simulink library "tp333079"  (Simulink 5.0)
values from neighbouring files (symbols this model uses):
  b = 1    [main_flock3.m]    (also in main_flock4.m; params_flocking_ros.m)
undefined symbols (not defined in the file or in its folder): AC, AlphaBnd, BetaBnd, CDda, CDde, CDdf, CDdr, CDM, CDmin, CGempty, CGgross, CL0, CLa, CLalphadot, Clbeta, Clda, CLde, CLdf, Cldr, CLM, CLmind, Clp, CLq, Clr, Cm0, Cma, Cmalphadot, Cmde, Cmdf, CmM, Cmq, Cnbeta, Cnda, Cndr, Cnp, Cnr, CP, CT, CYbeta, CYda, CYdr, CYp, CYr, Displacement, dmy, Engine, EulerIni, FuelFlow, FuelIni, J, Jempty, Jeng, Jgross, Jprop, MAC, MAP, MAPLim, MassIni, MaxPower, mempty ... (+26)
libraries: aerosimlib x325, simulink3 x42
(part 1 of 11)
Description:
  | AeroSim Aircraft Simulation Library
settings Model: Creator=Marius Niculescu  LastModifiedBy=mariusn

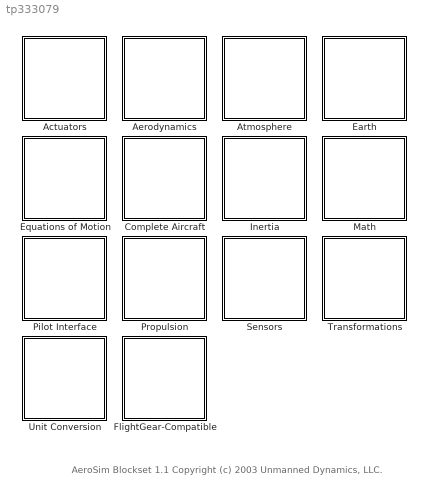
== system tp333079 ==
  note: AeroSim Blockset 1.1
      | Copyright (c) 2003 Unmanned Dynamics, LLC.
  Actuators : Subsystem  SimViewingDevice=off
      settings: Permissions=ReadWrite  RTWFcnNameOpts=Auto  RTWFileNameOpts=Auto
      mask Display: image(imread('act.bmp','bmp'))
  Aerodynamics : Subsystem  SimViewingDevice=off
      settings: Permissions=ReadWrite  RTWFcnNameOpts=Auto  RTWFileNameOpts=Auto
      mask Display: image(imread('aero.bmp','bmp'))
  Atmosphere : Subsystem  SimViewingDevice=off
      settings: Permissions=ReadWrite  RTWFcnNameOpts=Auto  RTWFileNameOpts=Auto
      mask Display: image(imread('atmo.bmp','bmp'))
  Complete Aircraft : Subsystem  SimViewingDevice=off
      settings: Permissions=ReadWrite  RTWFcnNameOpts=Auto  RTWFileNameOpts=Auto
      mask Display: image(imread('sample.bmp','bmp'))
  Earth : Subsystem  SimViewingDevice=off
      settings: Permissions=ReadWrite  RTWFcnNameOpts=Auto  RTWFileNameOpts=Auto
      mask Display: image(imread('earth.bmp','bmp'))
  Equations of Motion : Subsystem  SimViewingDevice=off
      settings: Permissions=ReadWrite  RTWFcnNameOpts=Auto  RTWFileNameOpts=Auto
      mask Display: image(imread('eom.bmp','bmp'))
  FlightGear-Compatible : Subsystem  SimViewingDevice=off
      settings: Permissions=ReadWrite  RTWFcnNameOpts=Auto  RTWFileNameOpts=Auto
      mask Display: image(imread('fg.bmp','bmp'))
  Inertia : Subsystem  SimViewingDevice=off
      settings: Permissions=ReadWrite  RTWFcnNameOpts=Auto  RTWFileNameOpts=Auto
      mask Display: image(imread('inertia.bmp','bmp'))
  Math : Subsystem  SimViewingDevice=off
      settings: Permissions=ReadWrite  RTWFcnNameOpts=Auto  RTWFileNameOpts=Auto
      mask Display: image(imread('linalg.bmp','bmp'))
  Pilot Interface : Subsystem  SimViewingDevice=off
      settings: Permissions=ReadWrite  RTWFcnNameOpts=Auto  RTWFileNameOpts=Auto
      mask Display: image(imread('pilot.bmp','bmp'))
  Propulsion : Subsystem  SimViewingDevice=off
      settings: Permissions=ReadWrite  RTWFcnNameOpts=Auto  RTWFileNameOpts=Auto
      mask Display: image(imread('prop.bmp','bmp'))
  Sensors : Subsystem  SimViewingDevice=off
      settings: Permissions=ReadWrite  RTWFcnNameOpts=Auto  RTWFileNameOpts=Auto
      mask Display: image(imread('sensor.bmp','bmp'))
  Transformations : Subsystem  SimViewingDevice=off
      settings: Permissions=ReadWrite  RTWFcnNameOpts=Auto  RTWFileNameOpts=Auto
      mask Display: image(imread('transf.bmp','bmp'))
  Unit Conversion : Subsystem  SimViewingDevice=off
      settings: Permissions=ReadWrite  RTWFcnNameOpts=Auto  RTWFileNameOpts=Auto
      mask Display: image(imread('units.bmp','bmp'))

== system tp333079/Actuators ==
  D/A Converter : Subsystem  SimViewingDevice=off  mask(D/A Converter){Vrange=[0 5], Bits=10, tsamp=0.02}
      mask prompts: Vrange "Voltage range [min max]:"; Bits "Resolution [bits]:"; tsamp "Sample time [s]:"
      mask help: Convert the digital signal with the specified resolution to analog voltage within a specified voltage range.
      mask init:
      | MinVolts = Vrange(1);
      | MaxVolts = Vrange(2);
      settings: Permissions=ReadWrite  RTWFcnNameOpts=Auto  RTWFileNameOpts=Auto
      mask Help:
      | <P>The D/A converter accepts a discrete signal as an integer number (counts) for input and provides an analog voltage. The parameters that have to be set are the following:</P>
      | <LI>Voltage range = a 1x2 vector with the minimum and maximum values of the output voltage;</LI>
      | <LI>Resolution = the maximum number of counts for input, i.e. a 10-bit converter can output maximum 2^10 = 1024 counts;</LI>
      | <LI>Sample time = input count update rate.</LI>
  Simple Actuator (1st-order dynamics) : Subsystem  SimViewingDevice=off  mask(Simple actuator){MaxRate=0.1, CountRange=[0 1024], ActRange=[-1 1], Lag=0.01}
      mask prompts: MaxRate "Max actuation rate:"; CountRange "Input signal range [min max]:"; ActRange "Actuator range [min max]:"; Lag "Actuator lag:"
      mask help: Simple actuator featuring 1st order dynamics, saturation and rate limits.
      mask init:
      | MinAct = ActRange(1); MaxAct = ActRange(2);
      | MinCounts = CountRange(1); MaxCounts = CountRange(2);
      settings: Permissions=ReadWrite  RTWFcnNameOpts=Auto  RTWFileNameOpts=Auto
      mask Help:
      | The block provides a simple actuator model which includes scaling, linear dynamics, saturation, and rate limits.
      | <P><B>Parameters:</B>
      | <LI>Maximum actuation rate = the max actuator travel speed, (travel per second)</LI>
      | <LI>Input signal range = the 1x2 vector which includes the min and max values of the input signal (for example, for a 10-bit analog output signal, the range would be [0 1023]).</LI>
      | <LI>Actuator range = the actuator travel range.</LI>
      | <LI>Actuator lag = the time lag of the actuator output.</LI>
      | </P>
  Simple Actuator (2nd-order dynamics) : Subsystem  SimViewingDevice=off  mask(Simple actuator){MaxRate=0.1, CountRange=[0 1024], ActRange=[-1 1], Bandwidth=100}
      mask prompts: MaxRate "Max actuation rate:"; CountRange "Input signal range [min max]:"; ActRange "Actuator range [min max]:"; Bandwidth "Bandwidth at -3dB [Hz]:"
      mask help: Simple actuator featuring 2nd order dynamics, saturation and rate limits.
      mask init:
      | MinAct = ActRange(1); MaxAct = ActRange(2);
      | MinCounts = CountRange(1); MaxCounts = CountRange(2);
      | wn = 2*pi*Bandwidth;
      | zeta = 0.5*10^(3/20);
      settings: Permissions=ReadWrite  RTWFcnNameOpts=Auto  RTWFileNameOpts=Auto
      mask Help:
      | The block provides a simple actuator model which includes scaling, linear dynamics, saturation, and rate limits.
      | <P><B>Parameters:</B>
      | <LI>Maximum actuation rate = the max actuator travel speed, (travel per second)</LI>
      | <LI>Input signal range = the 1x2 vector which includes the min and max values of the input signal (for example, for a 10-bit analog output signal, the range would be [0 1023]).</LI>
      | <LI>Actuator range = the actuator travel range.</LI>
      | <LI>Bandwidth at -3dB = the actuator bandwidth at -90 deg phase and -3dB gain.</LI>
      | </P>
  wires:
  Simple Actuator (2nd-order dynamics)/1(Output) -> ?

== system tp333079/Aerodynamics ==
  Aerodynamic Force : Subsystem  SimViewingDevice=off  mask(Aerodynamic force){S=S}
      mask prompts: S "Wing reference area:"
      mask help: Computes aerodynamic force in body axes.
      settings: Permissions=ReadWrite  RTWFcnNameOpts=Auto  RTWFileNameOpts=Auto
      mask Help:
      | The block computes the aerodynamic force in body axes.
      | <P><B>Inputs:</B>
      | <LI>CD = the coefficient of drag</LI>
      | <LI>CY = the coefficient of side force</LI>
      | <LI>CL = the coefficient of lift</LI>
      | <LI>pdyn = the dynamic pressure</LI>
      | <LI>WindAxesVel = the 3x1 vector of wind axes velocity components [Va beta alpha]'</LI>
      | </P>
      | <P><B>Output:</B> the 3x1 vector of aerodynamic forces in body axes</P>
      | <P><B>Parameters:</B>
      | <LI>S = the wing reference area</LI>
      | </P>
  Aerodynamic Moment : Subsystem  SimViewingDevice=off  mask(Aerodynamic moment){c=MAC, b=b, S=S}
      mask prompts: c "Mean aerodynamic chord:"; b "Wing span:"; S "Wing reference area:"
      mask help: Computes aerodynamic moment with respect to the aerodynamic center.
      settings: Permissions=ReadWrite  RTWFcnNameOpts=Auto  RTWFileNameOpts=Auto
      mask Help:
      | The block computes the aerodynamic moment with respect to the aerodynamic center.
      | <P><B>Inputs:</B>
      | <LI>Cl = the roll moment coefficient</LI>
      | <LI>Cm = the pitch moment coefficient</LI>
      | <LI>Cn = the yaw moment coefficient</LI>
      | </P>
      | <P><B>Output:</B> the 3x1 vector of aerodynamic moments about the aerodynamic center</P>
      | <P><B>Parameters:</B>
      | <LI>c = the mean aerodynamic chord</LI>
      | <LI>b = the reference wing span</LI>
      | <LI>S = the reference wing area</LI>
      | </P>
  Drag Coefficient : Subsystem  SimViewingDevice=off  mask(Drag coefficient){CL0=CLmind, CD0=CDmin, CDdf=CDdf, CDde=CDde, CDda=CDda, CDdr=CDdr, CDM=CDM, e=osw, b=b, S=S}
      mask prompts: CL0 "Lift at minimum drag (CL0):"; CD0 "Minimum drag (CD0):"; CDdf "Lift control derivative (CDdf):"; CDde "Pitch control derivative (CDde):"; CDda "Roll control derivative (CDda):"; CDdr "Yaw control derivative (CDdr):"; CDM "Mach number derivative (CDM):"; e "Oswald's coefficient (e):"; b "Wing span (b):"; S "Wing reference area (S):"
      mask help: Computes the drag coefficient by linear component build-up.
      mask init:
      | AR = b^2/S;
      | k = 1/(pi*AR*e);
      settings: Permissions=ReadWrite  RTWFcnNameOpts=Auto  RTWFileNameOpts=Auto
      mask Help:
      | The block computes the airplane drag coefficient using linear component build-up method.
      | <P><B>Inputs:</B>
      | <LI>WindAxesVel = the 3x1 vector of wind axes velocity components [Va beta alpha]'</LI>
      | <LI>Control = the 4x1 vector of aerodynamic controls [Flap Elevator Aileron Rudder]'</LI>
      | <LI>CL = the current coefficient of lift</LI>
      | <LI>Mach = the Mach number.</LI>
      | </P>
      | <P><B>Output:</B> the coefficient of drag CD.</P>
      | <P><B>Parameters:</B>
      | <LI>CL0 = CL at minimum drag</LI>
      | <LI>CD0 = minimum drag</LI>
      | <LI>CDdf = CD sensitivity to flap deflection</LI>
      | <LI>CDde = CD sensitivity to elevator deflection</LI>
      | <LI>CDda = CD sensitivity to aileron deflection</LI>
      | <LI>CDdr = CD sensitivity to rudder deflection</LI>
      | <LI>CDM = CD sensitivity to Mach number</LI>
      | <LI>e = the Oswald coefficient, for induced drag</LI>
      | <LI>b = the reference span</LI>
      | <LI>S = the reference area</LI>
      | </P>
  Dynamic Pressure : Subsystem  SimViewingDevice=off
      settings: Permissions=ReadWrite  RTWFcnNameOpts=Auto  RTWFileNameOpts=Auto
      mask Type: Dynamic pressure
      mask Description: Computes dynamic pressure based on current airspeed and air density.
      mask Help:
      | The block computes the dynamic pressure.
      | <P><B>Inputs:</B>
      | <LI>WindAxesVel = the 3x1 vector of wind axes velocity components [Va beta alpha]'</LI>
      | <LI>rho = the air density at current altitude</LI>
      | </P>
      | <P><B>Output:</B> Dynamic pressure.</P>
  Lift Coefficient : Subsystem  SimViewingDevice=off  mask(Lift coefficient){CL0=CL0, CLalpha=CLa, CLdf=CLdf, CLde=CLde, CLalphadot=CLalphadot, CLq=CLq, CLM=CLM, c=MAC}
      mask prompts: CL0 "Zero-alpha lift (CL0):"; CLalpha "alpha derivative (CLa):"; CLdf "Lift control derivative (CLdf):"; CLde "Pitch control derivative (CLde):"; CLalphadot "alpha_dot derivative (CLalphadot):"; CLq "Pitch rate derivative (CLq):"; CLM "Mach number derivative (CLM):"; c "Mean aerodynamic chord (c):"
      mask help: Computes lift coefficient using linear component build-up.
      settings: Permissions=ReadWrite  RTWFcnNameOpts=Auto  RTWFileNameOpts=Auto
      mask Help:
      | The block computes the airplane lift coefficient using linear component build-up method.
      | <P><B>Inputs:</B>
      | <LI>WindAxesVel = the 3x1 vector of wind axes velocity components [Va beta alpha]'</LI>
      | <LI>Control = the 4x1 vector of aerodynamic controls [Flap Elevator Aileron Rudder]'</LI>
      | <LI>AlphaBetaDot = the 2x1 vector of aerodynamic angle derivatives [dalpha/dt dbeta/dt]'</LI>
      | <LI>AngularRates = the 3x1 vector of body angular rates [p q r]'</LI>
      | <LI>Mach = the Mach number.</LI>
      | </P>
      | <P><B>Output:</B> the coefficient of lift CL.</P>
      | <P><B>Parameters:</B>
      | <LI>CL0 = CL at zero angle-of-attack</LI>
      | <LI>CLa = CL sensitivity to angle of attack</LI>
      | <LI>CLdf = CL sensitivity to flap deflection</LI>
      | <LI>CLde = CL sensitivity to elevator deflection</LI>
      | <LI>CLalphadot = CL sensitivity to time variations in angle of attack</LI>
      | <LI>CLq = CL sensitivity to pitch rate</LI>
      | <LI>CLM = CL sensitivity to Mach number</LI>
      | <LI>c = the reference chord (typically the mean aerodynamic chord of the wing)</LI>
      | </P>
  Pitch Moment Coefficient : Subsystem  SimViewingDevice=off  mask(Pitch moment coefficient){Cm0=Cm0, Cma=Cma, Cmdf=Cmdf, Cmde=Cmde, Cmalphadot=Cmalphadot, Cmq=Cmq, CmM=CmM, c=MAC}
      mask prompts: Cm0 "Zero-alpha pitch (Cm0):"; Cma "alpha derivative (Cma):"; Cmdf "Lift control derivative (Cmdf):"; Cmde "Pitch control derivative (Cmde):"; Cmalphadot "alpha_dot derivative (Cmalphadot):"; Cmq "Pitch rate derivative (Cmq):"; CmM "Mach number derivative (CmM):"; c "Mean aerodynamic chord (c):"
      mask help: Computes pitch moment coefficient using linear component build-up.
      settings: Permissions=ReadWrite  RTWFcnNameOpts=Auto  RTWFileNameOpts=Auto
      mask Help:
      | The block computes the airplane pitch moment coefficient using linear component build-up method.
      | <P><B>Inputs:</B>
      | <LI>WindAxesVel = the 3x1 vector of wind axes velocity components [Va beta alpha]'</LI>
      | <LI>Control = the 4x1 vector of aerodynamic controls [Flap Elevator Aileron Rudder]'</LI>
      | <LI>AlphaBetaDot = the 2x1 vector of aerodynamic angle derivatives [dalpha/dt dbeta/dt]'</LI>
      | <LI>AngularRates = the 3x1 vector of body angular rates [p q r]'</LI>
      | <LI>Mach = the Mach number.</LI>
      | </P>
      | <P><B>Output:</B> the pitch moment coefficient Cm.</P>
      | <P><B>Parameters:</B>
      | <LI>Cm0 = Cm at zero angle-of-attack</LI>
      | <LI>Cma = Cm sensitivity to angle of attack</LI>
      | <LI>Cmdf = Cm sensitivity to flap deflection</LI>
      | <LI>Cmde = Cm sensitivity to elevator deflection</LI>
      | <LI>Cmalphadot = Cm sensitivity to time variations in angle of attack</LI>
      | <LI>Cmq = Cm sensitivity to pitch rate</LI>
      | <LI>CmM = Cm sensitivity to Mach number</LI>
      | <LI>c = the reference chord (typically the mean aerodynamic chord of the wing)</LI>
      | </P>
  Roll Moment Coefficient : Subsystem  SimViewingDevice=off  mask(Roll moment coefficient){Clbeta=Clbeta, Clda=Clda, Cldr=Cldr, Clp=Clp, Clr=Clr, b=b}
      mask prompts: Clbeta "Sideslip derivative (Clbeta):"; Clda "Roll control derivative (Clda):"; Cldr "Yaw control derivative (Cldr):"; Clp "Roll rate derivative (Clp):"; Clr "Yaw rate derivative (Clr):"; b "Wing span (b):"
      mask help: Computes the roll moment coefficient using linear aerodynamic component build-up.
      settings: Permissions=ReadWrite  RTWFcnNameOpts=Auto  RTWFileNameOpts=Auto
      mask Help:
      | The block computes the airplane roll coefficient using linear component build-up method.
      | <P><B>Inputs:</B>
      | <LI>WindAxesVel = the 3x1 vector of wind axes velocity components [Va beta alpha]'</LI>
      | <LI>Control = the 4x1 vector of aerodynamic controls [Flap Elevator Aileron Rudder]'</LI>
      | <LI>AngularRates = the 3x1 vector of body angular rates [p q r]'</LI>
      | </P>
      | <P><B>Output:</B> the roll moment coefficient Cl.</P>
      | <P><B>Parameters:</B>
      | <LI>Clbeta = Cl sensitivity to sideslip</LI>
      | <LI>Clda = Cl sensitivity to aileron deflection</LI>
      | <LI>Cldr = Cl sensitivity to rudder deflection</LI>
      | <LI>Clp = Cl sensitivity to roll rate</LI>
      | <LI>Clr = Cl sensitivity to yaw rate</LI>
      | <LI>b = the reference wing span</LI>
      | </P>
  Side Force Coefficient : Subsystem  SimViewingDevice=off  mask(Side force coefficient){CYbeta=CYbeta, CYda=CYda, CYdr=CYdr, CYp=CYp, CYr=CYr, b=b}
      mask prompts: CYbeta "Sideslip derivative (CYbeta):"; CYda "Roll control derivative (CYda):"; CYdr "Yaw control derivative (CYdr):"; CYp "Roll rate derivative (CYp):"; CYr "Yaw rate derivative (CYr):"; b "Wing span (b):"
      mask help: Computes the side force coefficient using linear aerodynamic component build-up.
      settings: Permissions=ReadWrite  RTWFcnNameOpts=Auto  RTWFileNameOpts=Auto
      mask Help:
      | The block computes the airplane side force coefficient using linear component build-up method.
      | <P><B>Inputs:</B>
      | <LI>WindAxesVel = the 3x1 vector of wind axes velocity components [Va beta alpha]'</LI>
      | <LI>Control = the 4x1 vector of aerodynamic controls [Flap Elevator Aileron Rudder]'</LI>
      | <LI>AngularRates = the 3x1 vector of body angular rates [p q r]'</LI>
      | </P>
      | <P><B>Output:</B> the coefficient of side force CY.</P>
      | <P><B>Parameters:</B>
      | <LI>CYbeta = CY sensitivity to sideslip</LI>
      | <LI>CYda = CY sensitivity to aileron deflection</LI>
      | <LI>CYdr = CY sensitivity to rudder deflection</LI>
      | <LI>CYp = CY sensitivity to roll rate</LI>
      | <LI>CYr = CY sensitivity to yaw rate</LI>
      | <LI>b = the reference wing span</LI>
      | </P>
  Wind-axes Velocities : Subsystem  SimViewingDevice=off  mask(Wind-axes velocities){Vabnd=VaBnd, betabnd=BetaBnd, alphabnd=AlphaBnd}
      mask prompts: Vabnd "Airspeed bounds [min max]:"; betabnd "Sideslip angle bounds [min max]:"; alphabnd "Angle-of-attack bounds [min max]:"
      mask help: Returns the airspeed, sideslip angle, angle-of-attack and Mach number as functions of groundspeed, winds and local speed of sound. It also computes the time derivatives of the aerodynamic angles.
      settings: Permissions=ReadWrite  RTWFcnNameOpts=Auto  RTWFileNameOpts=Auto
      mask Help:
      | The block computes the wind-axes parameters including airspeed, angle-of-attack, and sideslip, as well as the wind angles time derivatives. In addition to that, the Mach number is computed.
      | <P><B>Inputs:</B>
      | <LI>Vbody = the 3x1 vector of body velocities (these are ground speed components in body axes)</LI>
      | <LI>Wbody = the 3x1 vector of wind velocities in body axes</LI>
      | <LI>SoundSpd = the speed of sound at current altitude</LI>
      | </P>
      | <P><B>Outputs:</B>
      | <LI>WindAxesVel = the 3x1 vector of wind-axes velocities [Va beta alpha]'</LI>
      | <LI>AlphaBetaDot = the 2x1 vector of angle derivatives [dalpha/dt dbeta/dt]'</LI>
      | <LI>Mach = the Mach number.</LI>
      | </P>
      | <P><B>Parameters:</B>
      | <LI> Airspeed bounds = the min and max allowed values of airspeed.</LI>
      | <LI>Sideslip angle bounds = the min and max values of allowed sideslip.</LI>
      | <LI>AOA bounds = the min and max values of allowed angle-of-attack.</LI>
      | <LI>These bound settings are provided such that the aircraft model does not exceed the flight regime for which aerodynamic data is available.</LI>
      | </P>
  Yaw Moment Coefficient : Subsystem  SimViewingDevice=off  mask(Yaw moment coefficient){Cnbeta=Cnbeta, Cnda=Cnda, Cndr=Cndr, Cnp=Cnp, Cnr=Cnr, b=b}
      mask prompts: Cnbeta "Sideslip derivative (Cnbeta):"; Cnda "Roll control derivative (Cnda):"; Cndr "Yaw control derivative (Cndr):"; Cnp "Roll rate derivative (Cnp):"; Cnr "Yaw rate derivative (Cnr):"; b "Wing span (b):"
      mask help: Computes the yaw moment coefficient using linear aerodynamic component build-up.
      settings: Permissions=ReadWrite  RTWFcnNameOpts=Auto  RTWFileNameOpts=Auto
      mask Help:
      | The block computes the airplane yaw moment coefficient using linear component build-up method.
      | <P><B>Inputs:</B>
      | <LI>WindAxesVel = the 3x1 vector of wind axes velocity components [Va beta alpha]'</LI>
      | <LI>Control = the 4x1 vector of aerodynamic controls [Flap Elevator Aileron Rudder]'</LI>
      | <LI>AngularRates = the 3x1 vector of body angular rates [p q r]'</LI>
      | </P>
      | <P><B>Output:</B> the yaw moment coefficient Cn.</P>
      | <P><B>Parameters:</B>
      | <LI>Cnbeta = Cn sensitivity to sideslip</LI>
      | <LI>Cnda = Cn sensitivity to aileron deflection</LI>
      | <LI>Cndr = Cn sensitivity to rudder deflection</LI>
      | <LI>Cnp = Cn sensitivity to roll rate</LI>
      | <LI>Cnr = Cn sensitivity to yaw rate</LI>
      | <LI>b = the reference wing span</LI>
      | </P>

== system tp333079/Atmosphere ==
  Background Wind : Subsystem  SimViewingDevice=off
      settings: Permissions=ReadWrite  RTWFcnNameOpts=Auto  RTWFileNameOpts=Auto
      mask Type: Background wind
      mask Description: Returns the background wind velocity and acceleration in body axes.
      mask Help:
      | The block computes the background wind velocity and acceleration in body axes, given the wind velocities in navigation frame, and the navigation-to-body frame transformation matrix.
      | <P><B>Inputs:</B>
      | <LI>WindsNED = the 3x1 vector of wind speed components  [North East Down]</LI>
      | <LI>DCM = the 3x3 frame transformation matrix, from navigation frame to body frame</LI>
      | </P>
      | <P><B>Output:</B>
      | <LI>WindVel = the 3x1 vector of wind speed components in body axes [x y z]</LI>
      | <LI>WindAcc = the 3x1 vector of wind accelerations in body axes.</LI>
      | </P>
  Standard Atmosphere : Subsystem  SimViewingDevice=off  mask(Standard atmosphere){}
      mask help: Compute standard atmosphere pressure, temperature, density and speed of sound as functions of MSL altitude.
      mask init:
      | load('stdatm');
      settings: Permissions=ReadWrite  RTWFcnNameOpts=Auto  RTWFileNameOpts=Auto
      mask Help:
      | The block computes the static pressure, temperature, density and speed of sound at current MSL altitude, using the 1976 Standard Atmosphere look-up tables.
      | <P><B>Inputs:</B>
      | <LI>MSLAlt = the altitude measured from mean-sea-level, in meters</LI>
      | </P>
      | <P><B>Output:</B>
      | <LI>p = the static pressure, in Pa</LI>
      | <LI>T = the outside air temperature, in K</LI>
      | <LI>rho = the air density, in kg/m^3</LI>
      | <LI>a = the speed of sound, in m/s</LI>
      | </P>
  Turbulence : Subsystem  SimViewingDevice=off  mask(Turbulence){tsamp=tsamp}
      mask prompts: tsamp "Sample time:"
      mask help: von Karman turbulence model returns turbulence velocity and acceleration in body axes.
      settings: Permissions=ReadWrite  RTWFcnNameOpts=Auto  RTWFileNameOpts=Auto
      mask Help:
      | The block provides von Karman turbulence models.
      | <P><B>Inputs:</B>
      | <LI>Wind-axes velocities = the 3x1 vector of aircraft velocities in wind axes [Airspeed Sideslip Angle-of-attack], in [m/s rad rad]</LI>
      | <LI>AGLAlt = the altitude of the aircraft above ground in m</LI>
      | <LI>WindVel = the 3x1 vector of background wind velocities in body axes</LI>
      | </P>
      | <P><B>Output:</B>
      | <LI>TurbVel = the 3x1 vector of turbulence wind components in body axes</LI>
      | <LI>TurbAcc = the 3x1 vector of turbulence acceleration components in body axes</LI>
      | </P>
      | <P><B>Parameters:</B>
      | <LI>Sample time = the sample time for turbulence filters</LI>
      | </P>
  Wind Shear : Subsystem  SimViewingDevice=off
      settings: Permissions=ReadWrite  RTWFcnNameOpts=Auto  RTWFileNameOpts=Auto
      mask Type: Wind shear
      mask Description: Computes the body angular rates due to wind and turbulence.
      mask Help:
      | The block computes the body angular rates due to wind and turbulence.
      | <P><B>Inputs:</B>
      | <LI>WindAcc = the background wind accelerations, in body axes</LI>
      | <LI>TurbAcc = the turbulence accelerations, in body axes</LI>
      | <LI>Velocities = the 3x1 vector of aircraft velocities in body axes</LI>
      | </P>
      | <P><B>Output:</B>
      | <LI>WindAngRates = the 3x1 vector of angular rates due to wind</LI>
      | <LI>WindAngAcc = the 3x1 vector of angular accelerations due to wind</LI>
      | </P>

== system tp333079/Complete Aircraft ==
  6-DOF Aircraft Model (Body-frame EOM) : Subsystem  SimViewingDevice=off  mask(6-DOF Aircraft Model){aircraftcfg='unknown.mat', VelocitiesIni=[0 0 0]', RatesIni=[0 0 0]', QuaternionsIni=[1 0 0 0]', PositionIni=[0*pi/180 0*pi/180 0]', FuelIni=0, OmegaIni=0*pi/30, GndAlt=0, wmmfile='c:\udynamics\projects\AeroSim\wmm.cof', dmy=[07 01 2002], tsamp=0.005}
      mask prompts: aircraftcfg "Aircraft configuration file:"; VelocitiesIni "Initial velocities:"; RatesIni "Initial angular rates:"; QuaternionsIni "Initial attitude:"; PositionIni "Initial position:"; FuelIni "Initial fuel mass:"; OmegaIni "Initial engine speed:"; GndAlt "Ground altitude:"; wmmfile "WMM coefficient file:"; dmy "Simulation date:"; tsamp "Sample time:"
      mask help: Nonlinear 6-DOF aircraft model with equations of motion in body frame.
      mask init:
      | load(aircraftcfg);
      settings: Permissions=ReadWrite  RTWFcnNameOpts=Auto  RTWFileNameOpts=Auto
      mask Help:
      | The block implements the 6-DOF nonlinear aircraft model using AeroSim blocks. Velocities are computed in body frame.
      | <P><B>Inputs:</B>
      | <LI>Controls = the 7x1 vector of aircraft controls [flap elevator aileron rudder throttle mixture ignition]. Aerodynamic controls are in radians, throttle is from 0 to 1, mixture is fraction air/fuel flow, ignition is 0 (engine off) or 1 (engine on).</LI>
      | <LI>Winds = the 3x1 vector of background wind speed components in navigation frame [North East Down]</LI>
      | <LI>RST = the integrator reset flag (0 or 1, all integrators on rising edge)
      | </P>
      | <P><B>Outputs:</B>
      | <LI>States = the 15x1 aircraft state vector [Velocities, Angular rates, Quaternions, Position, Fuel mass, Engine speed].</LI>
      | <LI>Sensors = the 18x1 vector of sensor outputs [GPS Position, GPS Groundspeed, Accelerometers, Gyros, Air data, Magnetometer].</LI>
      | <LI>VelW = the 3x1 vector of aircraft velocity in wind axes [Airspeed, sideslip, angle of attack]</LI>
      | <LI>Mach = the Mach number</LI>
      | <LI>Ang Acc = the 3x1 vector of angular accelerations
      | <LI>Euler = the 3x1 vector of Euler angles (roll, pitch, yaw)</LI>
      | <LI>AeroCoeff = the 6x1 vector of aerodynamic coefficients [CD CY CL Cl Cm Cn]</LI>
      | <LI>PropCoeff = the 3x1 vector of propeller coefficients [J CT CP]</LI>
      | <LI>EngCoeff = the 5x1 vector of engine coefficients [MAP Airflow Fuelflow BSFC Power]</LI>
      | <LI>Mass = the current aircraft mass</LI>
      | <LI>ECEF = 3x1 vector of position of the aircraft in the Earth-centered, Earth-fixed frame</LI>
      | <LI>MSL = the aircraft altitude above mean-sea-level</LI>
      | <LI>AGL = the aircraft altitude above terrain</LI>
      | <LI>REarth = the Earth equivalent radius at current location
      | <LI>AConGnd = the aircraft-on-ground flag (0 if aircraft above ground, 1 if aircraft on the ground)</LI>
      | </P>
      | <P><B>Parameters:</B>
      | <LI>Aircraft configuration file = the MAT-file with aircraft data</LI>
      | <LI>Initial velocities = the 3x1 vector of initial aircraft velocities in body axes [u v w]</LI>
      | <LI>Initial angular rates = the 3x1 vector of initial angular rates [p q r]</LI>
      | <LI>Initial attitude = the 4x1 vector of initial quaternions [e0 ex ey ez]</LI>
      | <LI>Initial position = the 3x1 vector of initial aircraft location [Lat Lon Alt]</LI>
      | <LI>Initial fuel mass = the initial quantity of fuel on-board the aircraft</LI>
      | <LI>Initial engine speed = the initial engine rotation speed</LI>
      | <LI>Ground altitude = the ground altitude at aircraft location</LI>
      | <LI>WMM coefficient file = the path to the magnetic model coefficient file</LI>
      | <LI>Simulation date = the date to be used for the magnetic model [day month year]</LI>
      | <LI>Sample time = the aircraft model sample time.</LI>
      | </P>
  6-DOF Aircraft Model (Geodetic-frame EOM) : Subsystem  SimViewingDevice=off  mask(6-DOF Aircraft Model){aircraftcfg='unknown.mat', PositionIni=[0*pi/180 0*pi/180 0]', VelocitiesIni=[0 0 0]', QuaternionsIni=[1 0 0 0]', RatesIni=[0 0 0]', FuelIni=0, OmegaIni=0*pi/30, GndAlt=0, wmmfile='c:\udynamics\projects\AeroSim\wmm.cof', dmy=[07 01 2002], tsamp=0.005}
      mask prompts: aircraftcfg "Aircraft configuration file:"; PositionIni "Initial position:"; VelocitiesIni "Initial velocities:"; QuaternionsIni "Initial attitude:"; RatesIni "Initial angular rates:"; FuelIni "Initial fuel mass:"; OmegaIni "Initial engine speed:"; GndAlt "Ground altitude:"; wmmfile "WMM coefficient file:"; dmy "Simulation date:"; tsamp "Sample time:"
      mask help: Nonlinear 6-DOF aircraft model with equations of motion in geodetic frame.
      mask init:
      | load(aircraftcfg);
      settings: Permissions=ReadWrite  RTWFcnNameOpts=Auto  RTWFileNameOpts=Auto
      mask Help:
      | The block implements the 6-DOF nonlinear aircraft model using AeroSim blocks. Velocity equations are implemented in geodetic frame. Angular rates take into account Earth's rotation speed.
      | <P><B>Inputs:</B>
      | <LI>Controls = the 7x1 vector of aircraft controls [flap elevator aileron rudder throttle mixture ignition]. Aerodynamic controls are in radians, throttle is from 0 to 1, mixture is fraction air/fuel flow, ignition is 0 (engine off) or 1 (engine on).</LI>
      | <LI>Winds = the 3x1 vector of background wind speed components in navigation frame [North East Down]</LI>
      | <LI>RST = the integrator reset flag (0 or 1, all integrators on rising edge)
      | </P>
      | <P><B>Outputs:</B>
      | <LI>States = the 15x1 aircraft state vector [Position, Velocity, Attitude (quaternions), Angular rates, Fuel mass, Engine speed].</LI>
      | <LI>Sensors = the 18x1 vector of sensor outputs [GPS Position, GPS Groundspeed, Accelerometers, Gyros, Air data, Magnetometer].</LI>
      | <LI>VelW = the 3x1 vector of aircraft velocity in wind axes [Airspeed, sideslip, angle of attack]</LI>
      | <LI>Mach = the Mach number</LI>
      | <LI>Ang Acc = the 3x1 vector of angular accelerations
      | <LI>Euler = the 3x1 vector of Euler angles (roll, pitch, yaw)</LI>
      | <LI>AeroCoeff = the 6x1 vector of aerodynamic coefficients [CD CY CL Cl Cm Cn]</LI>
      | <LI>PropCoeff = the 3x1 vector of propeller coefficients [J CT CP]</LI>
      | <LI>EngCoeff = the 5x1 vector of engine coefficients [MAP Airflow Fuelflow BSFC Power]</LI>
      | <LI>Mass = the current aircraft mass</LI>
      | <LI>ECEF = 3x1 vector of position of the aircraft in the Earth-centered, Earth-fixed frame</LI>
      | <LI>MSL = the aircraft altitude above mean-sea-level</LI>
      | <LI>AGL = the aircraft altitude above terrain</LI>
      | <LI>REarth = the Earth equivalent radius at aircraft location
      | <LI>AConGnd = the aircraft-on-ground flag (0 if aircraft above ground, 1 if aircraft on the ground)</LI>
      | </P>
      | <P><B>Parameters:</B>
      | <LI>Aircraft configuration file = the MAT-file with aircraft data</LI>
      | <LI>Initial position = the 3x1 vector of initial aircraft location [Lat Lon Alt]</LI>
      | <LI>Initial velocities = the 3x1 vector of initial aircraft velocities in geodetic frame [VN VE VD]</LI>
      | <LI>Initial attitude = the 4x1 vector of initial quaternions [e0 ex ey ez]</LI>
      | <LI>Initial angular rates = the 3x1 vector of initial angular rates [p q r]</LI>
      | <LI>Initial fuel mass = the initial quantity of fuel on-board the aircraft</LI>
      | <LI>Initial engine speed = the initial engine rotation speed</LI>
      | <LI>Ground altitude = the ground altitude at aircraft location</LI>
      | <LI>WMM coefficient file = the path to the magnetic model coefficient file</LI>
      | <LI>Simulation date = the date to be used for the magnetic model [day month year]</LI>
      | <LI>Sample time = the aircraft model sample time.</LI>
      | </P>
  6-DOF Aircraft Model (Geodetic-frame EOM) No magnetic field : Subsystem  SimViewingDevice=off  mask(6-DOF Aircraft Model){aircraftcfg='unknown.mat', PositionIni=[0*pi/180 0*pi/180 0]', VelocitiesIni=[0 0 0]', QuaternionsIni=[1 0 0 0]', RatesIni=[0 0 0]', FuelIni=0, OmegaIni=0*pi/30, GndAlt=0, tsamp=0.005}
      mask prompts: aircraftcfg "Aircraft configuration file:"; PositionIni "Initial position:"; VelocitiesIni "Initial velocities:"; QuaternionsIni "Initial attitude:"; RatesIni "Initial angular rates:"; FuelIni "Initial fuel mass:"; OmegaIni "Initial engine speed:"; GndAlt "Ground altitude:"; tsamp "Sample time:"
      mask help: Nonlinear 6-DOF aircraft model with equations of motion in geodetic frame.
      mask init:
      | load(aircraftcfg);
      settings: Permissions=ReadWrite  RTWFcnNameOpts=Auto  RTWFileNameOpts=Auto
      mask Help:
      | The block implements the 6-DOF nonlinear aircraft model using AeroSim blocks. Velocity equations are implemented in geodetic frame. Angular rates take into account Earth's rotation speed.
      | <P><B>Inputs:</B>
      | <LI>Controls = the 7x1 vector of aircraft controls [flap elevator aileron rudder throttle mixture ignition]. Aerodynamic controls are in radians, throttle is from 0 to 1, mixture is fraction air/fuel flow, ignition is 0 (engine off) or 1 (engine on).</LI>
      | <LI>Winds = the 3x1 vector of background wind speed components in navigation frame [North East Down]</LI>
      | <LI>RST = the integrator reset flag (0 or 1, all integrators on rising edge)
      | </P>
      | <P><B>Outputs:</B>
      | <LI>States = the 15x1 aircraft state vector [Position, Velocity, Attitude (quaternions), Angular rates, Fuel mass, Engine speed].</LI>
      | <LI>Sensors = the 18x1 vector of sensor outputs [GPS Position, GPS Groundspeed, Accelerometers, Gyros, Air data, Magnetometer].</LI>
      | <LI>VelW = the 3x1 vector of aircraft velocity in wind axes [Airspeed, sideslip, angle of attack]</LI>
      | <LI>Mach = the Mach number</LI>
      | <LI>Ang Acc = the 3x1 vector of angular accelerations
      | <LI>Euler = the 3x1 vector of Euler angles (roll, pitch, yaw)</LI>
      | <LI>AeroCoeff = the 6x1 vector of aerodynamic coefficients [CD CY CL Cl Cm Cn]</LI>
      | <LI>PropCoeff = the 3x1 vector of propeller coefficients [J CT CP]</LI>
      | <LI>EngCoeff = the 5x1 vector of engine coefficients [MAP Airflow Fuelflow BSFC Power]</LI>
      | <LI>Mass = the current aircraft mass</LI>
      | <LI>ECEF = 3x1 vector of position of the aircraft in the Earth-centered, Earth-fixed frame</LI>
      | <LI>MSL = the aircraft altitude above mean-sea-level</LI>
      | <LI>AGL = the aircraft altitude above terrain</LI>
      | <LI>REarth = the Earth equivalent radius at aircraft location
      | <LI>AConGnd = the aircraft-on-ground flag (0 if aircraft above ground, 1 if aircraft on the ground)</LI>
      | </P>
      | <P><B>Parameters:</B>
      | <LI>Aircraft configuration file = the MAT-file with aircraft data</LI>
      | <LI>Initial position = the 3x1 vector of initial aircraft location [Lat Lon Alt]</LI>
      | <LI>Initial velocities = the 3x1 vector of initial aircraft velocities in geodetic frame [VN VE VD]</LI>
      | <LI>Initial attitude = the 4x1 vector of initial quaternions [e0 ex ey ez]</LI>
      | <LI>Initial angular rates = the 3x1 vector of initial angular rates [p q r]</LI>
      | <LI>Initial fuel mass = the initial quantity of fuel on-board the aircraft</LI>
      | <LI>Initial engine speed = the initial engine rotation speed</LI>
      | <LI>Ground altitude = the ground altitude at aircraft location</LI>
      | <LI>Sample time = the aircraft model sample time.</LI>
      | </P>
  Glider Model : Subsystem  SimViewingDevice=off  mask(Glider model){aircraftcfg='unknown.mat', VelocitiesIni=[0 0 0]', RatesIni=[0 0 0]', QuaternionsIni=[1 0 0 0]', PositionIni=[0*pi/180 0*pi/180 0]', tsamp=0.005}
      mask prompts: aircraftcfg "Aircraft configuration file:"; VelocitiesIni "Initial velocities:"; RatesIni "Initial angular rates:"; QuaternionsIni "Initial attitude:"; PositionIni "Initial position:"; tsamp "Sample time:"
      mask help:
      | Simple un-powered model with equations of motion in body frame.
      | The model does not include propulsion, wind and turbulence effects, the Earth geoid and magnetic models. Also GPS-reported altitude coincides with the mean-sea-level altitude.
      mask init:
      | load(aircraftcfg);
      settings: Permissions=ReadWrite  RTWFcnNameOpts=Auto  RTWFileNameOpts=Auto
      mask Help:
      | Simple un-powered model with equations of motion in body frame.
      | The model does not include propulsion, wind and turbulence effects, the Earth geoid and magnetic models. Also GPS-reported altitude coincides with the mean-sea-level altitude.
      | <P><B>Inputs:</B>
      | <LI>Controls = the 4x1 vector of aerodynamic controls [flap elevator aileron rudder]. Aerodynamic controls are in radians.</LI>
      | </P>
      | <P><B>Outputs:</B>
      | <LI>States = the 13x1 aircraft state vector [Velocities, Angular rates, Quaternions, Position].</LI>
      | <LI>Sensors = the 15x1 vector of sensor outputs [GPS Position, GPS Groundspeed, Accelerometers, Gyros, Air data].</LI>
      | <LI>VelW = the 3x1 vector of aircraft velocity in wind axes [Airspeed, sideslip, angle of attack]</LI>
      | <LI>Mach = the Mach number</LI>
      | <LI>Ang Acc = the 3x1 vector of angular accelerations
      | <LI>Euler = the 3x1 vector of Euler angles (roll, pitch, yaw)</LI>
      | <LI>AeroCoeff = the 6x1 vector of aerodynamic coefficients [CD CY CL Cl Cm Cn]</LI>
      | </P>
      | <P><B>Parameters:</B>
      | <LI>Aircraft configuration file = the MAT-file with aircraft data</LI>
      | <LI>Initial velocities = the 3x1 vector of initial aircraft velocities in body axes [u v w]</LI>
      | <LI>Initial angular rates = the 3x1 vector of initial angular rates [p q r]</LI>
      | <LI>Initial attitude = the 4x1 vector of initial quaternions [e0 ex ey ez]</LI>
      | <LI>Initial position = the 3x1 vector of initial aircraft location [Lat Lon Alt]</LI>
      | <LI>Sample time = the aircraft model sample time.</LI>
      | </P>
  Inertial Navigation System : Subsystem  SimViewingDevice=off  mask(INS){PositionIni=[45*pi/180 -122*pi/180 1000]', VelocitiesIni=[23 0 1]', QuaternionsIni=[1 0 0 0]', tsamp=0.005}
      mask prompts: PositionIni "Initial position:"; VelocitiesIni "Initial velocities:"; QuaternionsIni "Initial attitude:"; tsamp "Sample time:"
      mask help: An Inertial Navigation System algorithm, using the geodetic-frame equations of motion.
      settings: Permissions=ReadWrite  RTWFcnNameOpts=Auto  RTWFileNameOpts=Auto
      mask Help:
      | An Inertial Navigation System algorithm, using the geodetic-frame equations of motion.
      | <P><B>Inputs:</B>
      | <LI>IMU = the 6x1 vector of inertial measurements, in body axes [accelerations, angular rates]
      | <LI>RST = the integrator reset flag (0 or 1, integrators resetting on rising edge)
      | </P>
      | <P><B>Outputs:</B>
      | <LI>PVA = the INS states [Position, Velocity, Attitude]
      | </P>
      | <P><B>Parameters:</B>
      | <LI>Initial position = the 3x1 vector of initial position [Lat Lon Alt]
      | <LI>Initial velocities = the 3x1 vector of initial velocities in geodetic frame [VN VE VD]
      | <LI>Initial attitude = the 4x1 vector of initial quaternions [e0 ex ey ez]
      | <LI>Sample time = the INS sample time.
      | </P>
  Simple Aircraft Model : Subsystem  SimViewingDevice=off  mask(Simple Aircraft Model){aircraftcfg='unknown.mat', VelocitiesIni=[0 0 0]', RatesIni=[0 0 0]', QuaternionsIni=[1 0 0 0]', PositionIni=[0*pi/180 0*pi/180 0]', FuelIni=0, OmegaIni=0*pi/30, tsamp=0.005}
      mask prompts: aircraftcfg "Aircraft configuration file:"; VelocitiesIni "Initial velocities:"; RatesIni "Initial angular rates:"; QuaternionsIni "Initial attitude:"; PositionIni "Initial position:"; FuelIni "Initial fuel mass:"; OmegaIni "Initial engine speed:"; tsamp "Sample time:"
      mask help:
      | Simple nonlinear 6-DOF aircraft model with equations of motion in body frame.
      | The model does not include wind and turbulence effects, the Earth geoid and magnetic models. Also GPS-reported altitude coincides with the mean-sea-level altitude.
      mask init:
      | load(aircraftcfg);
      settings: Permissions=ReadWrite  RTWFcnNameOpts=Auto  RTWFileNameOpts=Auto
      mask Help:
      | Simple nonlinear 6-DOF aircraft model with equations of motion in body frame.
      | The model does not include wind and turbulence effects, the Earth geoid and magnetic models. Also GPS-reported altitude coincides with the mean-sea-level altitude.
      | <P><B>Inputs:</B>
      | <LI>Controls = the 7x1 vector of aircraft controls [flap elevator aileron rudder throttle mixture ignition]. Aerodynamic controls are in radians, throttle is from 0 to 1, mixture is fraction air/fuel flow, ignition is 0 (engine off) or 1 (engine on).</LI>
      | </P>
      | <P><B>Outputs:</B>
      | <LI>States = the 15x1 aircraft state vector [Velocities, Angular rates, Quaternions, Position, Fuel mass, Engine speed].</LI>
      | <LI>Sensors = the 15x1 vector of sensor outputs [GPS Position, GPS Groundspeed, Accelerometers, Gyros, Air data].</LI>
      | <LI>VelW = the 3x1 vector of aircraft velocity in wind axes [Airspeed, sideslip, angle of attack]</LI>
      | <LI>Mach = the Mach number</LI>
      | <LI>Ang Acc = the 3x1 vector of angular accelerations
      | <LI>Euler = the 3x1 vector of Euler angles (roll, pitch, yaw)</LI>
      | <LI>AeroCoeff = the 6x1 vector of aerodynamic coefficients [CD CY CL Cl Cm Cn]</LI>
      | <LI>PropCoeff = the 3x1 vector of propeller coefficients [J CT CP]</LI>
      | <LI>EngCoeff = the 5x1 vector of engine coefficients [MAP Airflow Fuelflow BSFC Power]</LI>
      | <LI>Mass = the current aircraft mass</LI>
      | </P>
      | <P><B>Parameters:</B>
      | <LI>Aircraft configuration file = the MAT-file with aircraft data</LI>
      | <LI>Initial velocities = the 3x1 vector of initial aircraft velocities in body axes [u v w]</LI>
      | <LI>Initial angular rates = the 3x1 vector of initial angular rates [p q r]</LI>
      | <LI>Initial attitude = the 4x1 vector of initial quaternions [e0 ex ey ez]</LI>
      | <LI>Initial position = the 3x1 vector of initial aircraft location [Lat Lon Alt]</LI>
      | <LI>Initial fuel mass = the initial quantity of fuel on-board the aircraft</LI>
      | <LI>Initial engine speed = the initial engine rotation speed</LI>
      | <LI>Sample time = the aircraft model sample time.</LI>
      | </P>

== system tp333079/Earth ==
  EGM-96 : Subsystem  SimViewingDevice=off  mask(EGM-96 geoid undulation model){}
      mask help: The geoid undulation model computes the MSL (mean sea level) altitude as a function of position.
      mask init:
      | load('egm96');
      settings: Permissions=ReadWrite  RTWFcnNameOpts=Auto  RTWFileNameOpts=Auto
      mask Help:
      | The block computes the mean-sea-level altitude relative to the WGS-84 geoid.
      | <P><B>Inputs:</B>
      | <LI>Position = the 3x1 vector of aircraft location [Latitude Longitude Altitude], in [rad rad m]</LI>
      | </P>
      | <P><B>Output:</B>
      | <LI>MSLAlt = the mean-sea-level altitude, in m</LI>
      | </P>
  Ground Detection : Subsystem  SimViewingDevice=off
      settings: Permissions=ReadWrite  RTWFcnNameOpts=Auto  RTWFileNameOpts=Auto
      mask Type: Ground detection
      mask Description: Computes altitude above ground and sets a flag if AGL is negative.
      mask Help:
      | The block computes the altitude above ground (AGL) and sets a flag if the AGL is negative (used for ground contact detection).
      | <P><B>Inputs:</B>
      | <LI>MSLAlt = the altitude measured from mean-sea-level, in meters</LI>
      | <LI>GndAlt = the altitude of the terrain (above MSL) at current location, in meters</LI>
      | </P>
      | <P><B>Output:</B>
      | <LI>AConGnd = the aircraft-on-ground flag (0 if aircraft above ground, 1 if aircraft on the ground)</LI>
      | <LI>AGLAlt = the altitude of the aircraft above ground</LI>
      | </P>
  WGS-84 : Subsystem  SimViewingDevice=off
      settings: Permissions=ReadWrite  RTWFcnNameOpts=Auto  RTWFileNameOpts=Auto
      mask Type: WGS-84 Earth model
      mask Description: The WGS-84 Earth model provides local Earth radii and gravity as a function of position.
      mask Help:
      | The block provides a WGS-84 geoid model of the Earth.
      | <P><B>Inputs:</B>
      | <LI>Position = current aircraft location [Latitude Longitude Altitude], in [rad rad m]</LI>
      | </P>
      | <P><B>Output:</B>
      | <LI>Rmeridian = the Earth meridian radius, in m</LI>
      | <LI>Rnormal = the Earth normal radius, in m</LI>
      | <LI>Re = the Earth equivalent radius, in m</LI>
      | <LI>Gravity = the normal gravity, in m/s^2</LI>
      | </P>
  WMM-2000 : Subsystem  SimViewingDevice=off  mask(WMM-2000){wmmfile='c:\udynamics\projects\AeroSim\wmm.cof', simdate=dmy}
      mask prompts: wmmfile "WMM coefficient file:"; simdate "Simulation date [Day Month Year]:"
      mask help: The World Magnetic Model returns the Earth magnetic field components in body axes at current aircraft location.
      settings: Permissions=ReadWrite  RTWFcnNameOpts=Auto  RTWFileNameOpts=Auto
      mask Help:
      | The block provides the magnetic field components at current aircraft location.
      | <P><B>Inputs:</B>
      | <LI>Position = the 3x1 vector of aircraft location [Latitude Longitude Altitude] in [rad rad m]</LI>
      | <LI>DCM = the frame transformation matrix from navigation to body frame</LI>
      | </P>
      | <P><B>Output:</B>
      | <LI>MagField = the 3x1 vector of magnetic field components in body axes</LI>
      | </P>
      | <P><B>Parameters:</B>
      | <LI>WMM coefficient file = the path to the WMM coefficient file, as a 'string'</LI>
      | <LI>Simulation date = the 1x3 vector of current date [Day Month Year]</LI>
      | </P>

== system tp333079/Equations of Motion ==
  Body-Frame EOM : Subsystem  SimViewingDevice=off
      settings: Permissions=ReadWrite  RTWFcnNameOpts=Auto  RTWFileNameOpts=Auto
  Geodetic-Frame EOM : Subsystem  SimViewingDevice=off
      settings: Permissions=ReadWrite  RTWFcnNameOpts=Auto  RTWFileNameOpts=Auto
  Total Acceleration : Subsystem  SimViewingDevice=off
      settings: Permissions=ReadWrite  RTWFcnNameOpts=Auto  RTWFileNameOpts=Auto
      mask Type: Total acceleration
      mask Description: Computes total airframe acceleration as a sum of aerodynamic and propulsion forces.
      mask Help:
      | The block computes the total acceleration applied to the airframe due to aerodynamics and propulsion.
      | <P><B>Inputs:</B>
      | <LI> 3x1 vector of aerodynamic forces;</LI>
      | <LI> 3x1 vector of propulsion forces;</LI>
      | <LI> current aircraft mass;</LI>
      | </P>
      | <P><B>Outputs:</B>
      | <LI> 3x1 vector of accelerations in body frame;</LI>
      | </P>
  Total Moment : Subsystem  SimViewingDevice=off  mask(Total moment){raero=rAC, rprop=rHub}
      mask prompts: raero "Aerodynamic force application point:"; rprop "Propulsion force application point:"
      mask help: Compute the total airframe moment with respect to the current CG location.
      settings: Permissions=ReadWrite  RTWFcnNameOpts=Auto  RTWFileNameOpts=Auto
      mask Help:
      | The block computes the total moment applied to the airframe with respect to the current CG location. The forces that generate moment about CG are the aerodynamics and the propulsion.
      | <P><B>Parameters:</B>
      | <LI> 3x1 position vector from origin to the aerodynamic forces application point;</LI>
      | <LI> 3x1 position vector from origin to the propulsion forces application point;</LI>
      | </P>
      | <P><B>Inputs:</B>
      | <LI> 3x1 vector of aerodynamic forces;</LI>
      | <LI> 3x1 vector of aerodynamic moments;</LI>
      | <LI> 3x1 vector of propulsion forces;</LI>
      | <LI> 3x1 vector of propulsion moments;</LI>
      | <LI> 3x1 vector of position from origin to current CG location;</LI>
      | </P>
      | <P><B>Output:</B> 3x1 vector of moments about the CG.</P>

== system tp333079/FlightGear-Compatible ==
  Aerodynamics : Subsystem  SimViewingDevice=off
      settings: Permissions=ReadWrite  RTWFcnNameOpts=Auto  RTWFileNameOpts=Auto
      mask Display: image(imread('aero.bmp','bmp'))
  Complete Aircraft : Subsystem  SimViewingDevice=off
      settings: Permissions=ReadWrite  RTWFcnNameOpts=Auto  RTWFileNameOpts=Auto
      mask Display: image(imread('sample.bmp','bmp'))
  Inertia : Subsystem  SimViewingDevice=off
      settings: Permissions=ReadWrite  RTWFcnNameOpts=Auto  RTWFileNameOpts=Auto
      mask Display: image(imread('inertia.bmp','bmp'))
  Propulsion : Subsystem  SimViewingDevice=off
      settings: Permissions=ReadWrite  RTWFcnNameOpts=Auto  RTWFileNameOpts=Auto
      mask Display: image(imread('prop.bmp','bmp'))
